simulink model "LinearFurnace"  (R2019a)
settings: Solver=VariableStepAuto  StartTime=0.0  StopTime=5000  RelTol=1e-3
undefined symbols (not defined in the file or in its folder): A_O2_aI, A_O2_aII, A_O2_grate, A_O2_w, A_st_aI, A_st_aII, A_st_grate, A_st_w, aI_step, aII_step, B_st_aI, B_st_aII, B_st_grate, C_O2_grate, C_st_aI, F_O2_offset, F_st_offset, grate_step, reg, T12_st_aI, T12_st_aII, T12_st_grate, T1_O2_aI, T1_O2_aII, T1_O2_grate, T1_O2_w, T1_st_aII, T1_st_w, T2_st_aI, T2_st_grate, T3_O2_grate, T3_st_aI, w_step
libraries: simulink x3
settings Model: Creator=hermanko  LastModifiedBy=hermanko
settings DataIOCC: FinalStateName=state_final  InitialState=state_init_lin2  LoadInitialState=on  SaveFinalState=on  SaveOperatingPoint=on  SaveState=on

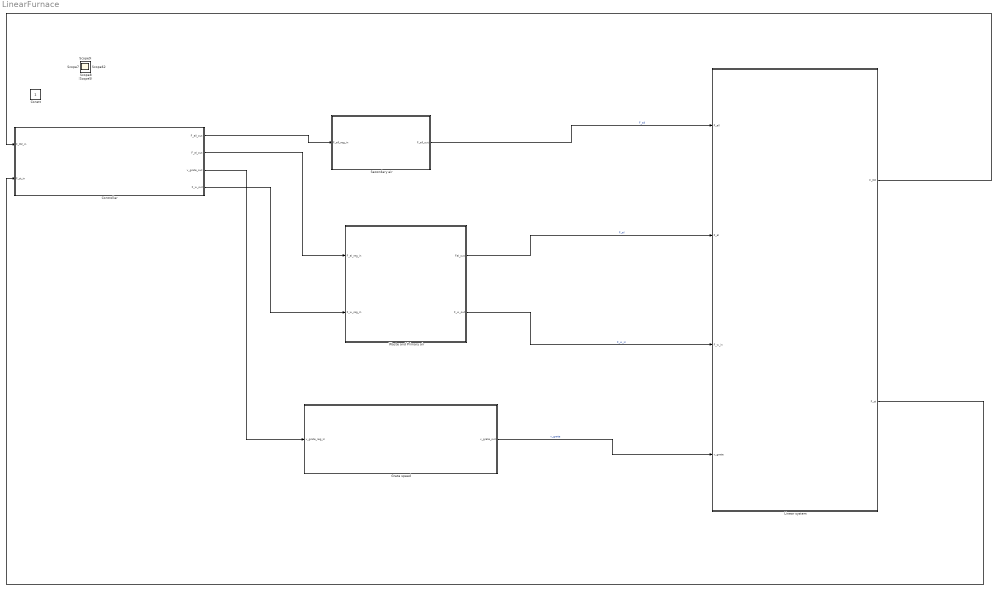
== system LinearFurnace ==
  Controller : Subsystem
  Grate speed : Subsystem
  Linear system : Subsystem
  Secondary air : Subsystem
      mask Display: image('airflow.jpeg');
  Waste and Primary air : Subsystem
      mask Display: image('waste_in.jpg');
  Constt : Constant  IOType=siggen
  Scope{,1..10,12} (12 alike) : Scope
  wires:
  Controller/1(F_aII_out) -> Secondary air/1(F_aII_reg_in)
  Controller/2(F_aI_out) -> Waste and Primary air/1("F_aI_reg_in ")
  Controller/4(F_w_out) -> Waste and Primary air/2(F_w_reg_in)
  Controller/3(v_grate_out) -> Grate speed/1(v_grate_reg_in)
  Linear system/1(F_O2) -> Controller/1(F_O2_in)
  Linear system/2(F_st) -> Controller/2(F_st_in)
  Secondary air/1(F_aII_out) -> Linear system/1(F_aII)  "F_aII"
  Waste and Primary air/1(FaI_out) -> Linear system/2(F_aI)  "F_aI"
  Waste and Primary air/2(F_w_out) -> Linear system/3(F_w_in)  "F_w_in"
  Grate speed/1(v_grate_out) -> Linear system/4(v_grate)  "v_grate"

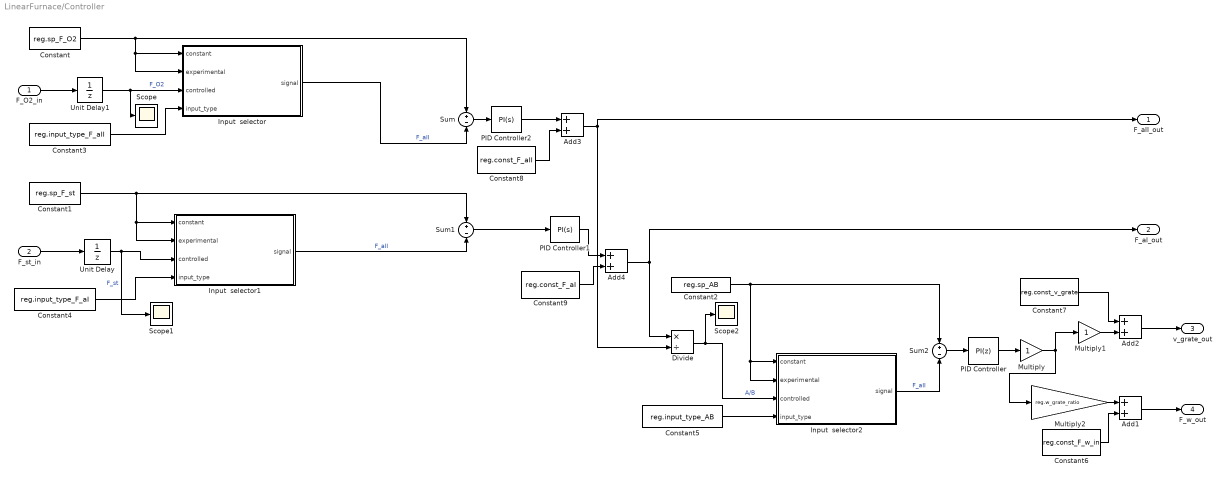
== system LinearFurnace/Controller ==
  F_O2_in : Inport
  F_st_in : Inport  Port=2
  Add{1..4} (4 alike) : Sum
  Constant : Constant  Value=reg.sp_F_O2
  Constant1 : Constant  Value=reg.sp_F_st
  Constant2 : Constant  Value=reg.sp_AB
  Constant3 : Constant  Value=reg.input_type_F_aII
  Constant4 : Constant  Value=reg.input_type_F_aI
  Constant5 : Constant  Value=reg.input_type_AB
  Constant6 : Constant  Value=reg.const_F_w_in
  Constant7 : Constant  Value=reg.const_v_grate
  Constant8 : Constant  Value=reg.const_F_aII
  Constant9 : Constant  Value=reg.const_F_aI
  Divide : Product  Inputs=*/  OutMin=[-100]  OutMax=[100]
  Input  selector : MATLAB Function  TreatAsAtomicUnit=on
  Input  selector1 : MATLAB Function  TreatAsAtomicUnit=on
  Input  selector2 : MATLAB Function  TreatAsAtomicUnit=on
  Multiply : Gain
  Multiply1 : Gain
  Multiply2 : Gain  Gain=reg.w_grate_ratio
  PID Controller : simulink/Continuous/PID Controller  Controller=PI  Form=Parallel  TimeDomain=Discrete-time  SampleTime=-1  IntegratorMethod=Forward Euler  FilterMethod=Forward Euler  ControllerParametersSource=internal  P=reg.Kp_AB  I=reg.Ki_AB  D=0  UseFilter=on  N=100  TunerSelectOption=Transfer Function Based (PID Tuner App)  InitialConditionSource=internal  InitialConditionForIntegrator=0  InitialConditionForFilter=0  DifferentiatorICPrevScaledInput=0  ExternalReset=none  TrackingMode=off  Kt=1  LimitOutput=off  UpperSaturationLimit=inf  LowerSaturationLimit=-inf  LinearizeAsGain=on  AntiWindupMode=none  Kb=1  POutMin=[]  POutMax=[]  IOutMin=[]  IOutMax=[]  DOutMin=[]  DOutMax=[]  NOutMin=[]  NOutMax=[]  SumOutMin=[]  SumOutMax=[]  SaturationOutMin=[]  SaturationOutMax=[]  PParamMin=[]  PParamMax=[]  IParamMin=[]  IParamMax=[]  DParamMin=[]  DParamMax=[]  NParamMin=[]  NParamMax=[]  KbParamMin=[]  KbParamMax=[]  KtParamMin=[]  KtParamMax=[]  KbOutMin=[]  KbOutMax=[]  KtOutMin=[]  KtOutMax=[]  IntegratorOutMin=[]  IntegratorOutMax=[]  FilterOutMin=[]  FilterOutMax=[]  SumI1OutMin=[]  SumI1OutMax=[]  SumI2OutMin=[]  SumI2OutMax=[]  SumI3OutMin=[]  SumI3OutMax=[]  SumI4OutMin=[]  SumI4OutMax=[]  SumDOutMin=[]  SumDOutMax=[]  DifferentiatorOutMin=[]  DifferentiatorOutMax=[]  FilterDiffOutCoefMin=[]  FilterDiffOutCoefMax=[]  ReciprocalOutMin=[]  ReciprocalOutMax=[]  SumDenOutMin=[]  SumDenOutMax=[]  SumNumOutMin=[]  SumNumOutMax=[]  DivideOutMin=[]  DivideOutMax=[]  IntegratorContinuousStateAttributes=''  IntegratorStateMustResolveToSignalObject=off  IntegratorRTWStateStorageClass=Auto  FilterContinuousStateAttributes=''  FilterStateMustResolveToSignalObject=off  FilterRTWStateStorageClass=Auto  ParallelPVariant=InternalParameters  IdealPVariant=Disabled  IVariant=InternalParameters  DVariant=Disabled  IntegratorVariant=Discrete  SatVariant=Disabled  AWVariant=Passthrough  PCopyVariant=Disabled  TRVariant=Disabled  FdbkBlocksVariant=Forward  IdealPFdbkVariant=Disabled  SatFdbkVariant=Disabled  DerivativeFilterVariant=Disabled  NVariant=Disabled  NCopyVariant=Disabled_SignalSpec  FilterICVariant=Disabled  IntegratorICVariant=InternalICs  ExternalResetVariant=Disabled  TRSumVariant=Passthrough  SumFdbkVariant=Disabled  SumVariant=Sum_PI
  PID Controller1 : simulink/Continuous/PID Controller  Controller=PI  Form=Parallel  TimeDomain=Continuous-time  SampleTime=-1  IntegratorMethod=Forward Euler  FilterMethod=Forward Euler  ControllerParametersSource=internal  P=reg.Kp_st  I=reg.Ki_st  D=0  UseFilter=on  N=100  TunerSelectOption=Transfer Function Based (PID Tuner App)  InitialConditionSource=internal  InitialConditionForIntegrator=0  InitialConditionForFilter=0  DifferentiatorICPrevScaledInput=0  ExternalReset=none  TrackingMode=off  Kt=1  LimitOutput=off  UpperSaturationLimit=inf  LowerSaturationLimit=1  LinearizeAsGain=on  AntiWindupMode=none  Kb=1  POutMin=[]  POutMax=[]  IOutMin=[]  IOutMax=[]  DOutMin=[]  DOutMax=[]  NOutMin=[]  NOutMax=[]  SumOutMin=[]  SumOutMax=[]  SaturationOutMin=[]  SaturationOutMax=[]  PParamMin=[]  PParamMax=[]  IParamMin=[]  IParamMax=[]  DParamMin=[]  DParamMax=[]  NParamMin=[]  NParamMax=[]  KbParamMin=[]  KbParamMax=[]  KtParamMin=[]  KtParamMax=[]  KbOutMin=[]  KbOutMax=[]  KtOutMin=[]  KtOutMax=[]  IntegratorOutMin=[]  IntegratorOutMax=[]  FilterOutMin=[]  FilterOutMax=[]  SumI1OutMin=[]  SumI1OutMax=[]  SumI2OutMin=[]  SumI2OutMax=[]  SumI3OutMin=[]  SumI3OutMax=[]  SumI4OutMin=[]  SumI4OutMax=[]  SumDOutMin=[]  SumDOutMax=[]  DifferentiatorOutMin=[]  DifferentiatorOutMax=[]  FilterDiffOutCoefMin=[]  FilterDiffOutCoefMax=[]  ReciprocalOutMin=[]  ReciprocalOutMax=[]  SumDenOutMin=[]  SumDenOutMax=[]  SumNumOutMin=[]  SumNumOutMax=[]  DivideOutMin=[]  DivideOutMax=[]  IntegratorContinuousStateAttributes='F_st'  IntegratorStateMustResolveToSignalObject=off  IntegratorRTWStateStorageClass=Auto  FilterContinuousStateAttributes=''  FilterStateMustResolveToSignalObject=off  FilterRTWStateStorageClass=Auto  ParallelPVariant=InternalParameters  IdealPVariant=Disabled  IVariant=InternalParameters  DVariant=Disabled  IntegratorVariant=Continuous  SatVariant=Disabled  AWVariant=Passthrough  PCopyVariant=Disabled  TRVariant=Disabled  FdbkBlocksVariant=Forward  IdealPFdbkVariant=Disabled  SatFdbkVariant=Disabled  DerivativeFilterVariant=Disabled  NVariant=Disabled  NCopyVariant=Disabled_SignalSpec  FilterICVariant=Disabled  IntegratorICVariant=InternalICs  ExternalResetVariant=Disabled  TRSumVariant=Passthrough  SumFdbkVariant=Disabled  SumVariant=Sum_PI
  PID Controller2 : simulink/Continuous/PID Controller  Controller=PI  Form=Parallel  TimeDomain=Continuous-time  SampleTime=-1  IntegratorMethod=Forward Euler  FilterMethod=Forward Euler  ControllerParametersSource=internal  P=reg.Kp_O2  I=reg.Ki_O2  D=0  UseFilter=on  N=100  TunerSelectOption=Transfer Function Based (PID Tuner App)  InitialConditionSource=internal  InitialConditionForIntegrator=0.0000001  InitialConditionForFilter=0  DifferentiatorICPrevScaledInput=0  ExternalReset=none  TrackingMode=off  Kt=1  LimitOutput=off  UpperSaturationLimit=inf  LowerSaturationLimit=1  LinearizeAsGain=on  AntiWindupMode=none  Kb=1  POutMin=[]  POutMax=[]  IOutMin=[]  IOutMax=[]  DOutMin=[]  DOutMax=[]  NOutMin=[]  NOutMax=[]  SumOutMin=[]  SumOutMax=[]  SaturationOutMin=[]  SaturationOutMax=[]  PParamMin=[]  PParamMax=[]  IParamMin=[]  IParamMax=[]  DParamMin=[]  DParamMax=[]  NParamMin=[]  NParamMax=[]  KbParamMin=[]  KbParamMax=[]  KtParamMin=[]  KtParamMax=[]  KbOutMin=[]  KbOutMax=[]  KtOutMin=[]  KtOutMax=[]  IntegratorOutMin=[]  IntegratorOutMax=[]  FilterOutMin=[]  FilterOutMax=[]  SumI1OutMin=[]  SumI1OutMax=[]  SumI2OutMin=[]  SumI2OutMax=[]  SumI3OutMin=[]  SumI3OutMax=[]  SumI4OutMin=[]  SumI4OutMax=[]  SumDOutMin=[]  SumDOutMax=[]  DifferentiatorOutMin=[]  DifferentiatorOutMax=[]  FilterDiffOutCoefMin=[]  FilterDiffOutCoefMax=[]  ReciprocalOutMin=[]  ReciprocalOutMax=[]  SumDenOutMin=[]  SumDenOutMax=[]  SumNumOutMin=[]  SumNumOutMax=[]  DivideOutMin=[]  DivideOutMax=[]  IntegratorContinuousStateAttributes='F_st'  IntegratorStateMustResolveToSignalObject=off  IntegratorRTWStateStorageClass=Auto  FilterContinuousStateAttributes=''  FilterStateMustResolveToSignalObject=off  FilterRTWStateStorageClass=Auto  ParallelPVariant=InternalParameters  IdealPVariant=Disabled  IVariant=InternalParameters  DVariant=Disabled  IntegratorVariant=Continuous  SatVariant=Disabled  AWVariant=Passthrough  PCopyVariant=Disabled  TRVariant=Disabled  FdbkBlocksVariant=Forward  IdealPFdbkVariant=Disabled  SatFdbkVariant=Disabled  DerivativeFilterVariant=Disabled  NVariant=Disabled  NCopyVariant=Disabled_SignalSpec  FilterICVariant=Disabled  IntegratorICVariant=InternalICs  ExternalResetVariant=Disabled  TRSumVariant=Passthrough  SumFdbkVariant=Disabled  SumVariant=Sum_PI
  Scope : Scope
  Scope1 : Scope
  Scope2 : Scope
  Sum : Sum  Inputs=+|-
  Sum1 : Sum  Inputs=+|-
  Sum2 : Sum  Inputs=+|-
  Unit Delay : UnitDelay  HasFrameUpgradeWarning=on
  Unit Delay1 : UnitDelay  SampleTime=-1  HasFrameUpgradeWarning=on
  F_aII_out : Outport
  F_aI_out : Outport  Port=2
  v_grate_out : Outport  Port=3
  F_w_out : Outport  Port=4
  wires:
  Constant1/1 -> Input  selector1/2(experimental), Input  selector1/1(constant), Sum1/1
  F_st_in/1 -> Unit Delay/1
  Constant/1 -> Input  selector/1(constant), Input  selector/2(experimental), Sum/1
  Constant2/1 -> Input  selector2/2(experimental), Input  selector2/1(constant), Sum2/1
  F_O2_in/1 -> Unit Delay1/1
  Input  selector1/1(signal) -> Sum1/2  "F_aII"
  Input  selector/1(signal) -> Sum/2  "F_aII"
  Constant3/1 -> Input  selector/4(input_type)
  Constant4/1 -> Input  selector1/4(input_type)
  Constant5/1 -> Input  selector2/4(input_type)
  Divide/1 -> Scope2/1, Input  selector2/3(controlled)  "A/B"
  Input  selector2/1(signal) -> Sum2/2  "F_aII"
  Sum/1 -> PID Controller2/1
  Sum1/1 -> PID Controller1/1
  Sum2/1 -> PID Controller/1
  PID Controller/1 -> Multiply/1
  Unit Delay/1 -> Scope1/1, Input  selector1/3(controlled)  "F_st"
  Unit Delay1/1 -> Scope/1, Input  selector/3(controlled)  "F_O2"
  Multiply/1 -> Multiply2/1, Multiply1/1
  Multiply2/1 -> Add1/1
  Constant6/1 -> Add1/2
  Add1/1 -> F_w_out/1
  Add2/1 -> v_grate_out/1
  Multiply1/1 -> Add2/2
  Constant7/1 -> Add2/1
  Constant8/1 -> Add3/2
  PID Controller1/1 -> Add4/1
  PID Controller2/1 -> Add3/1
  Constant9/1 -> Add4/2
  Add3/1 -> F_aII_out/1, Divide/2
  Add4/1 -> F_aI_out/1, Divide/1

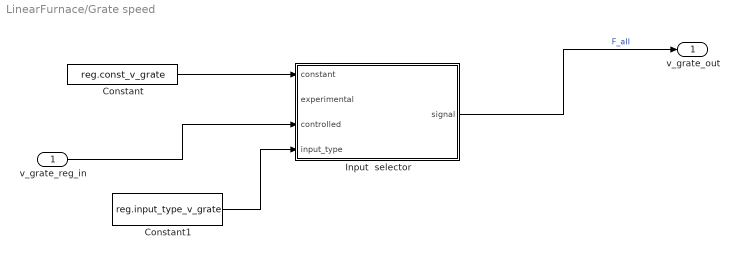
== system LinearFurnace/Grate speed ==
  v_grate_reg_in : Inport
  Constant : Constant  Value=reg.const_v_grate
  Constant1 : Constant  Value=reg.input_type_v_grate
  Input  selector : MATLAB Function  TreatAsAtomicUnit=on
  v_grate_out : Outport
  wires:
  Constant/1 -> Input  selector/1(constant)
  v_grate_reg_in/1 -> Input  selector/3(controlled)
  Constant1/1 -> Input  selector/4(input_type)
  Input  selector/1(signal) -> v_grate_out/1  "F_aII"

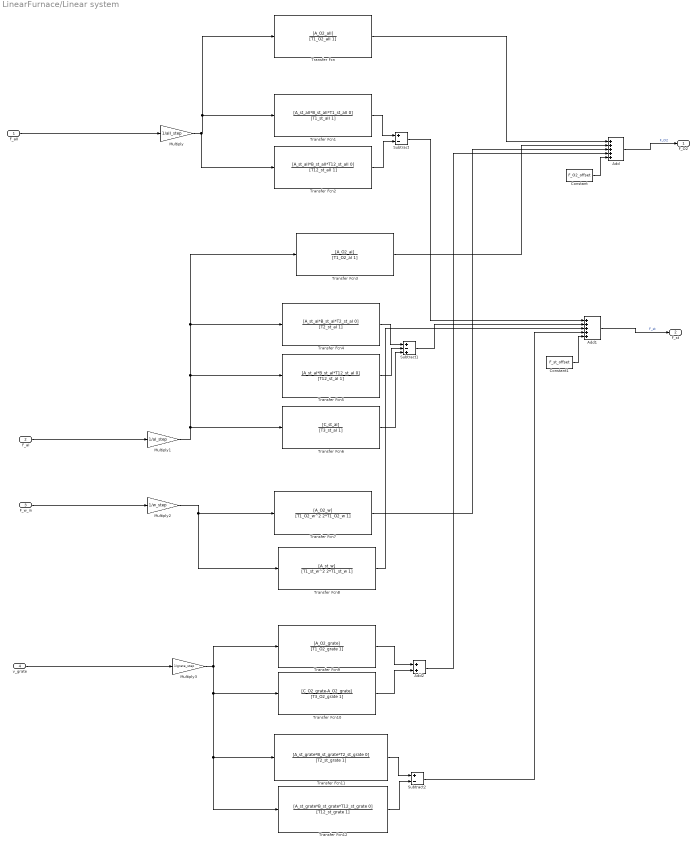
== system LinearFurnace/Linear system ==
  F_aII : Inport
  F_aI : Inport  Port=2
  F_w_in : Inport  Port=3
  v_grate : Inport  Port=4
  Add : Sum  Inputs=+++++
  Add1 : Sum  Inputs=+++++
  Add2 : Sum
  Constant : Constant  Value=F_O2_offset
  Constant1 : Constant  Value=F_st_offset
  Multiply : Gain  Gain=1/aII_step
  Multiply1 : Gain  Gain=1/aI_step
  Multiply2 : Gain  Gain=1/w_step
  Multiply3 : Gain  Gain=1/grate_step
  Subtract : Sum  Inputs=+-
  Subtract1 : Sum  Inputs=+-+
  Subtract2 : Sum  Inputs=+-
  Transfer Fcn : TransferFcn  Numerator=[A_O2_aII]  Denominator=[T1_O2_aII 1]
  Transfer Fcn1 : TransferFcn  Numerator=[A_st_aII*B_st_aII*T1_st_aII 0]  Denominator=[T1_st_aII 1]
  Transfer Fcn10 : TransferFcn  Numerator=[C_O2_grate-A_O2_grate]  Denominator=[T3_O2_grate 1]
  Transfer Fcn11 : TransferFcn  Numerator=[A_st_grate*B_st_grate*T2_st_grate 0]  Denominator=[T2_st_grate 1]
  Transfer Fcn12 : TransferFcn  Numerator=[A_st_grate*B_st_grate*T12_st_grate 0]  Denominator=[T12_st_grate 1]
  Transfer Fcn2 : TransferFcn  Numerator=[A_st_aII*B_st_aII*T12_st_aII 0]  Denominator=[T12_st_aII 1]
  Transfer Fcn3 : TransferFcn  Numerator=[A_O2_aI]  Denominator=[T1_O2_aI 1]
  Transfer Fcn4 : TransferFcn  Numerator=[A_st_aI*B_st_aI*T2_st_aI 0]  Denominator=[T2_st_aI 1]
  Transfer Fcn5 : TransferFcn  Numerator=[A_st_aI*B_st_aI*T12_st_aI 0]  Denominator=[T12_st_aI 1]
  Transfer Fcn6 : TransferFcn  Numerator=[C_st_aI]  Denominator=[T3_st_aI 1]
  Transfer Fcn7 : TransferFcn  Numerator=[A_O2_w]  Denominator=[T1_O2_w^2 2*T1_O2_w 1]
  Transfer Fcn8 : TransferFcn  Numerator=[A_st_w]  Denominator=[T1_st_w^2 2*T1_st_w 1]
  Transfer Fcn9 : TransferFcn  Numerator=[A_O2_grate]  Denominator=[T1_O2_grate 1]
  F_O2 : Outport
  F_st : Outport  Port=2
  wires:
  Transfer Fcn10/1 -> Add2/2
  Transfer Fcn2/1 -> Subtract/2
  Subtract/1 -> Add1/1
  Transfer Fcn6/1 -> Subtract1/3
  Transfer Fcn4/1 -> Subtract1/1
  Multiply2/1 -> Transfer Fcn8/1, Transfer Fcn7/1
  F_aI/1 -> Multiply1/1
  Transfer Fcn3/1 -> Add/2
  Transfer Fcn9/1 -> Add2/1
  Transfer Fcn5/1 -> Subtract1/2
  Multiply1/1 -> Transfer Fcn4/1, Transfer Fcn3/1, Transfer Fcn5/1, Transfer Fcn6/1
  Add1/1 -> F_st/1  "F_st"
  Transfer Fcn11/1 -> Subtract2/1
  Multiply3/1 -> Transfer Fcn12/1, Transfer Fcn11/1, Transfer Fcn10/1, Transfer Fcn9/1
  Subtract2/1 -> Add1/4
  Transfer Fcn8/1 -> Add1/3
  F_w_in/1 -> Multiply2/1
  Constant/1 -> Add/5
  Transfer Fcn7/1 -> Add/3
  Constant1/1 -> Add1/5
  Multiply/1 -> Transfer Fcn2/1, Transfer Fcn/1, Transfer Fcn1/1
  Add2/1 -> Add/4
  v_grate/1 -> Multiply3/1
  Transfer Fcn/1 -> Add/1
  Subtract1/1 -> Add1/2
  Transfer Fcn1/1 -> Subtract/1
  Transfer Fcn12/1 -> Subtract2/2
  F_aII/1 -> Multiply/1
  Add/1 -> F_O2/1  "F_O2"

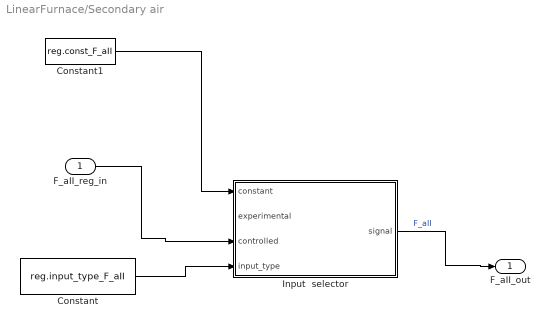
== system LinearFurnace/Secondary air ==
  F_aII_reg_in : Inport
  Constant : Constant  Value=reg.input_type_F_aII
  Constant1 : Constant  Value=reg.const_F_aII
  Input  selector : MATLAB Function  TreatAsAtomicUnit=on
  F_aII_out : Outport
  wires:
  Input  selector/1(signal) -> F_aII_out/1  "F_aII"
  F_aII_reg_in/1 -> Input  selector/3(controlled)
  Constant1/1 -> Input  selector/1(constant)
  Constant/1 -> Input  selector/4(input_type)

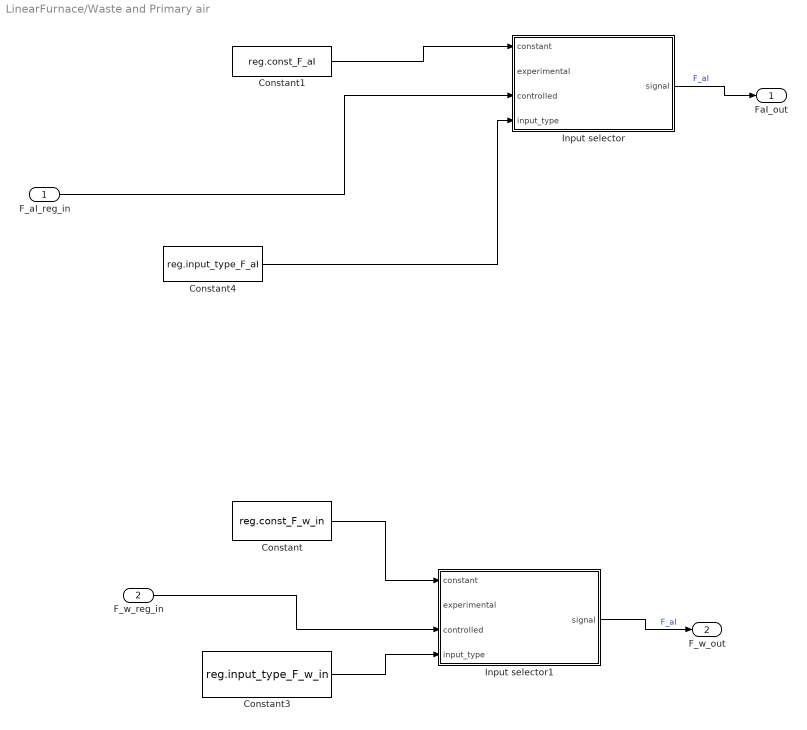
== system LinearFurnace/Waste and Primary air ==
  "F_aI_reg_in " : Inport
  F_w_reg_in : Inport  Port=2
  Constant : Constant  Value=reg.const_F_w_in
  Constant1 : Constant  Value=reg.const_F_aI
  Constant3 : Constant  Value=reg.input_type_F_w_in
  Constant4 : Constant  Value=reg.input_type_F_aI
  Input selector : MATLAB Function  TreatAsAtomicUnit=on
  Input selector1 : MATLAB Function  TreatAsAtomicUnit=on
  FaI_out : Outport
  F_w_out : Outport  Port=2
  wires:
  Constant/1 -> Input selector1/1(constant)
  Input selector/1(signal) -> FaI_out/1  "F_aI"
  "F_aI_reg_in "/1 -> Input selector/3(controlled)
  Constant1/1 -> Input selector/1(constant)
  Constant4/1 -> Input selector/4(input_type)
  Input selector1/1(signal) -> F_w_out/1  "F_aI"
  Constant3/1 -> Input selector1/4(input_type)
  F_w_reg_in/1 -> Input selector1/3(controlled)

== matlab function LinearFurnace/Waste and Primary air/Input selector1 ==
  data: constant input; signal output; experimental input; controlled input; input_type input
function signal = ChooseSignal(constant, experimental, controlled, input_type)
    switch(input_type)
        case InputType.Experimental
            signal = experimental;
        case InputType.Controlled
            signal = controlled;
        otherwise
            signal = constant;
    end
end

== matlab function LinearFurnace/Grate speed/Input  selector ==
  data: constant input; signal output; experimental input; controlled input; input_type input
function signal = ChooseSignal(constant, experimental, controlled, input_type)
    switch(input_type)
        case InputType.Experimental
            signal = experimental;
        case InputType.Controlled
            signal = controlled;
        otherwise
            signal = constant;
    end
end

== matlab function LinearFurnace/Controller/Input  selector ==
  data: constant input; signal output; experimental input; controlled input; input_type input
function signal = ChooseSignal(constant, experimental, controlled, input_type)
    switch(input_type)
        case InputType.Experimental
            signal = experimental;
        case InputType.Controlled
            signal = controlled;
        otherwise
            signal = constant;
    end
end

== matlab function LinearFurnace/Controller/Input  selector1 ==
  data: constant input; signal output; experimental input; controlled input; input_type input
function signal = ChooseSignal(constant, experimental, controlled, input_type)
    switch(input_type)
        case InputType.Experimental
            signal = experimental;
        case InputType.Controlled
            signal = controlled;
        otherwise
            signal = constant;
    end
end

== matlab function LinearFurnace/Controller/Input  selector2 ==
  data: constant input; signal output; experimental input; controlled input; input_type input
function signal = ChooseSignal(constant, experimental, controlled, input_type)
    switch(input_type)
        case InputType.Experimental
            signal = experimental;
        case InputType.Controlled
            signal = controlled;
        otherwise
            signal = constant;
    end
end

== matlab function LinearFurnace/Waste and Primary air/Input selector ==
  data: constant input; signal output; experimental input; controlled input; input_type input
function signal = ChooseSignal(constant, experimental, controlled, input_type)
    switch(input_type)
        case InputType.Experimental
            signal = experimental;
        case InputType.Controlled
            signal = controlled;
        otherwise
            signal = constant;
    end
end

== matlab function LinearFurnace/Secondary air/Input  selector ==
  data: constant input; signal output; experimental input; controlled input; input_type input
function signal = ChooseSignal(constant, experimental, controlled, input_type)
    switch(input_type)
        case InputType.Experimental
            signal = experimental;
        case InputType.Controlled
            signal = controlled;
        otherwise
            signal = constant;
    end
end
